simulink library "winch001_cl"  (R2022a)
settings: Solver=VariableStepAuto  StartTime=0.0  StopTime=10.0  RelTol=1e-3
undefined symbols (not defined in the file): firstOrderFilter, firstOrderFilter_ul, wnch
settings Model: Creator=jcreed2  LastModifiedBy=lhill8
settings SolverCC: AlgebraicLoopSolver=TrustRegion
settings DebuggingCC: UnconnectedInputMsg=warning  UnconnectedOutputMsg=warning  UnconnectedLineMsg=warning  SFMachineParentedDataDiag=warning  ArithmeticOperatorsInVariantConditions=warning
settings SFSimCC: CustomCodeUndefinedFunction=UseInterfaceOnly

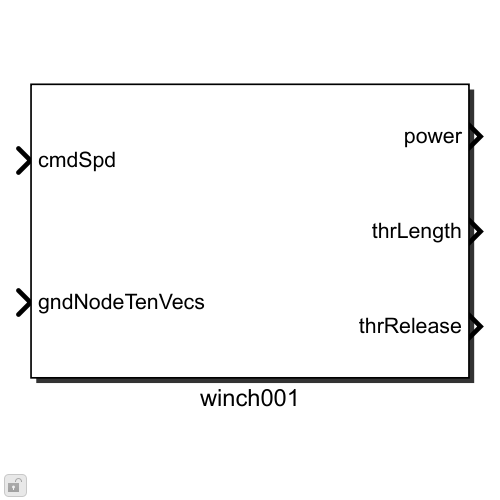
[thumbnail: Simulink's stored preview of the top-level diagram]
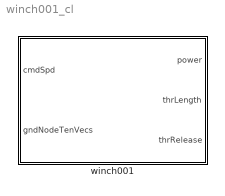
== system winch001_cl ==
  winch001 : Subsystem  VariantControl=VSS_winch_winch001

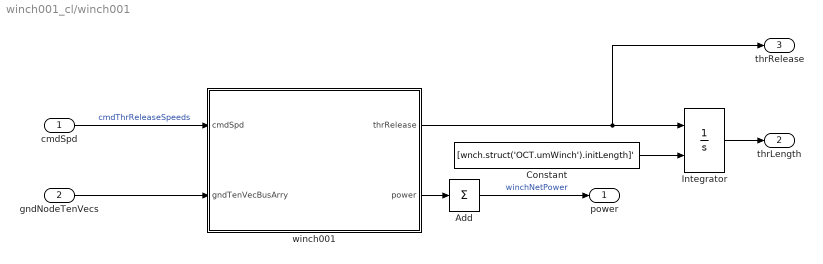
== system winch001_cl/winch001 ==
  cmdSpd : Inport
  gndNodeTenVecs : Inport  Port=2
  Add : Sum  Inputs=+
  Constant : Constant  Value=[wnch.struct('OCT.umWinch').initLength]'  VectorParams1D=off
  Integrator : Integrator  InitialConditionSource=external
  winch001 : Subsystem  mask{wnchStrct=wnch.struct('OCT.umWinch')}
      mask prompts: wnchStrct "Winch Structure"
  power : Outport  VectorParamsAs1DForOutWhenUnconnected=off
  thrLength : Outport  Port=2  VectorParamsAs1DForOutWhenUnconnected=off
  thrRelease : Outport  Port=3  VectorParamsAs1DForOutWhenUnconnected=off
  wires:
  winch001/1(thrRelease) -> Integrator/1, thrRelease/1
  Integrator/1 -> thrLength/1
  Constant/1 -> Integrator/2
  Add/1 -> power/1  "winchNetPower"
  winch001/2(power) -> Add/1
  gndNodeTenVecs/1 -> winch001/2(gndTenVecBusArry)
  cmdSpd/1 -> winch001/1(cmdSpd)  "cmdThrReleaseSpeeds"

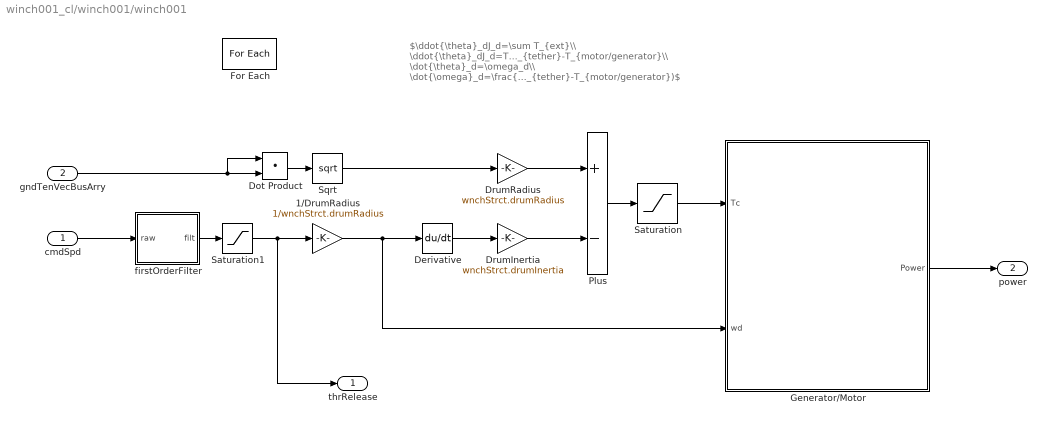
== system winch001_cl/winch001/winch001 ==
  note: $\ddot{\theta}_dJ_d=\sum T_{ext}\\ \ddot{\theta}_dJ_d=T_{tether}-T_{motor/generator}\\ \dot{\theta}_d=\omega_d\\ \dot{\omega}_d=\frac{1}{J_d}(T_{tether}-T_{motor/generator})$
  cmdSpd : Inport  Partition=on  PartitionDimension=1  PartitionWidth=1  PartitionOffset=0
  gndTenVecBusArry : Inport  Port=2  Partition=on  PartitionDimension=3  PartitionWidth=1  PartitionOffset=0
  1/DrumRadius : Gain  Gain=1/wnchStrct.drumRadius
  Derivative : Derivative
  Dot Product : DotProduct  OutDataTypeStr=Inherit: Inherit via internal rule
  DrumInertia : Gain  Gain=wnchStrct.drumInertia
  DrumRadius : Gain  Gain=wnchStrct.drumRadius
  For Each : ForEach  DisableCoverage=on  IterateSubsysMaskParameter=on  SubsysMaskParameterIterationDimension=2
  Generator/Motor : Subsystem
  Plus : Sum  Inputs=+-
  Saturation : Saturate  UpperLimit=inf  LowerLimit=0
  Saturation1 : Saturate  UpperLimit=wnchStrct.maxSpeed  LowerLimit=-wnchStrct.maxSpeed  LinearizeAsGain=off
  Sqrt : Sqrt
  firstOrderFilter : Subsystem  AncestorBlock=firstOrderFilter_ul/firstOrderFilter  TreatAsAtomicUnit=on  mask{tau=wnchStrct.timeConst, ic=wnchStrct.initReleaseRate}
      mask prompts: tau "Time Const [s]"; ic "Initial Condition"
      settings: MinAlgLoopOccurrences=on
  thrRelease : Outport  ConcatenationDimension=1  VectorParamsAs1DForOutWhenUnconnected=off
  power : Outport  Port=2  ConcatenationDimension=1  VectorParamsAs1DForOutWhenUnconnected=off
  wires:
  DrumInertia/1 -> Plus/2
  Derivative/1 -> DrumInertia/1
  DrumRadius/1 -> Plus/1
  Sqrt/1 -> DrumRadius/1
  Saturation1/1 -> 1/DrumRadius/1, thrRelease/1
  gndTenVecBusArry/1 -> Dot Product/2, Dot Product/1
  Dot Product/1 -> Sqrt/1
  Saturation/1 -> Generator/Motor/1(Tc)
  cmdSpd/1 -> firstOrderFilter/1(raw)
  1/DrumRadius/1 -> Generator/Motor/2(wd), Derivative/1
  Plus/1 -> Saturation/1
  Generator/Motor/1(Power) -> power/1
  firstOrderFilter/1(filt) -> Saturation1/1

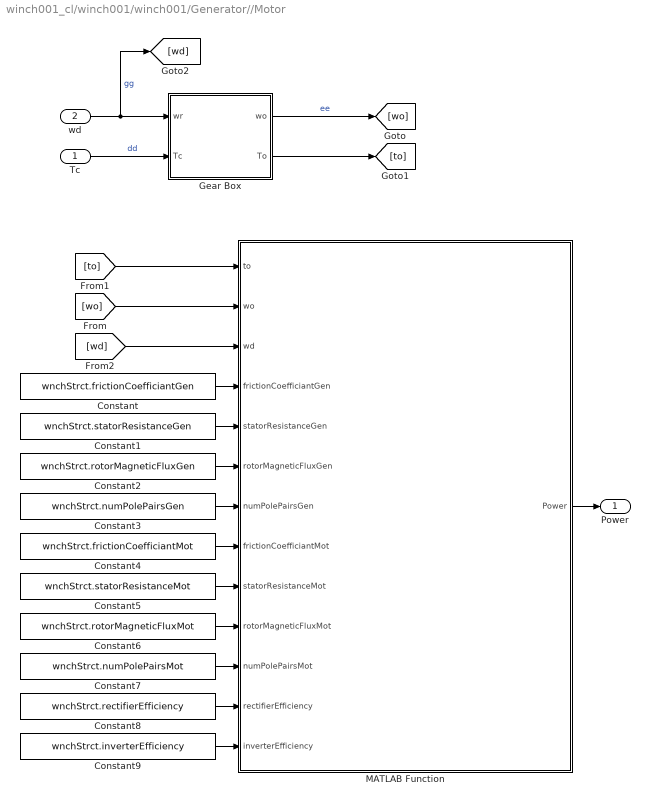
== system winch001_cl/winch001/winch001/Generator//Motor ==
  Tc : Inport
  wd : Inport  Port=2
  Constant : Constant  Value=wnchStrct.frictionCoefficiantGen
  Constant1 : Constant  Value=wnchStrct.statorResistanceGen
  Constant2 : Constant  Value=wnchStrct.rotorMagneticFluxGen
  Constant3 : Constant  Value=wnchStrct.numPolePairsGen
  Constant4 : Constant  Value=wnchStrct.frictionCoefficiantMot
  Constant5 : Constant  Value=wnchStrct.statorResistanceMot
  Constant6 : Constant  Value=wnchStrct.rotorMagneticFluxMot
  Constant7 : Constant  Value=wnchStrct.numPolePairsMot
  Constant8 : Constant  Value=wnchStrct.rectifierEfficiency
  Constant9 : Constant  Value=wnchStrct.inverterEfficiency
  Gear Box : Subsystem  mask{gfb=wnchStrct.gearRatio, Np=wnchStrct.numOfGearPairs}
      mask prompts: gfb "Gear Ratio"; Np "Number of Gear Pairs"
  MATLAB Function : MATLAB Function  TreatAsAtomicUnit=on
  Power : Outport  VectorParamsAs1DForOutWhenUnconnected=off
  wires:
  [wd] -> MATLAB Function/3(wd)
  [to] -> MATLAB Function/1(to)
  [wo] -> MATLAB Function/2(wo)
  Gear Box/2(To) -> [to]
  Gear Box/1(wo) -> [wo]  "ee"
  MATLAB Function/1(Power) -> Power/1
  Constant9/1 -> MATLAB Function/13(inverterEfficiency)
  Constant8/1 -> MATLAB Function/12(rectifierEfficiency)
  Constant7/1 -> MATLAB Function/11(numPolePairsMot)
  Constant6/1 -> MATLAB Function/10(rotorMagneticFluxMot)
  Constant5/1 -> MATLAB Function/9(statorResistanceMot)
  Constant4/1 -> MATLAB Function/8(frictionCoefficiantMot)
  Constant3/1 -> MATLAB Function/7(numPolePairsGen)
  Constant2/1 -> MATLAB Function/6(rotorMagneticFluxGen)
  Constant1/1 -> MATLAB Function/5(statorResistanceGen)
  Constant/1 -> MATLAB Function/4(frictionCoefficiantGen)
  wd/1 -> Gear Box/1(wr), [wd]  "gg"
  Tc/1 -> Gear Box/2(Tc)  "dd"

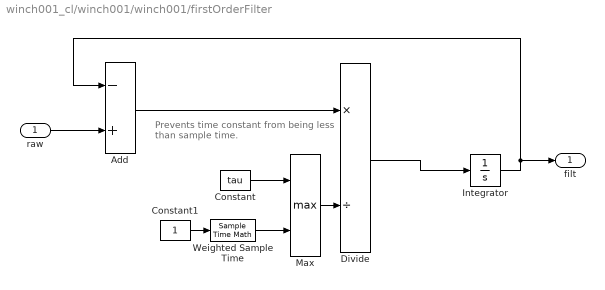
== system winch001_cl/winch001/winch001/firstOrderFilter ==
  note: Prevents time constant from
      | being less than sample time.
  raw : Inport
  Add : Sum  Inputs=-+
  Constant : Constant  Value=tau
  Constant1 : Constant
  Divide : Product  Inputs=*/
  Integrator : Integrator  InitialCondition=ic
  Max : MinMax  Function=max  Inputs=2
  Weighted Sample Time : SampleTimeMath  TsampMathOp=Ts Only
  filt : Outport  VectorParamsAs1DForOutWhenUnconnected=off
  wires:
  raw/1 -> Add/2
  Add/1 -> Divide/1
  Max/1 -> Divide/2
  Constant/1 -> Max/1
  Constant1/1 -> Weighted Sample Time/1
  Weighted Sample Time/1 -> Max/2
  Divide/1 -> Integrator/1
  Integrator/1 -> Add/1, filt/1

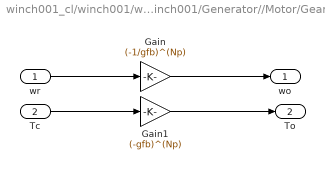
== system winch001_cl/winch001/winch001/Generator//Motor/Gear Box ==
  wr : Inport
  Tc : Inport  Port=2
  Gain : Gain  Gain=(-1/gfb)^(Np)
  Gain1 : Gain  Gain=(-gfb)^(Np)
  wo : Outport  VectorParamsAs1DForOutWhenUnconnected=off
  To : Outport  Port=2  VectorParamsAs1DForOutWhenUnconnected=off
  wires:
  wr/1 -> Gain/1
  Gain/1 -> wo/1
  Tc/1 -> Gain1/1
  Gain1/1 -> To/1

== matlab function winch001_cl/winch001/winch001/Generator//Motor/MATLAB Function ==
  data: to input; Power output; wo input; wd input; frictionCoefficiantGen input; statorResistanceGen input; rotorMagneticFluxGen input; numPolePairsGen input; frictionCoefficiantMot input; statorResistanceMot input; rotorMagneticFluxMot input; numPolePairsMot input; rectifierEfficiency input; inverterEfficiency input
function Power = fcn(to,wo,wd,frictionCoefficiantGen,statorResistanceGen,rotorMagneticFluxGen,numPolePairsGen,frictionCoefficiantMot,statorResistanceMot,rotorMagneticFluxMot,numPolePairsMot,rectifierEfficiency,inverterEfficiency)


Power = 0;

switch sign(wd)
    case 1
        
        wdAbs = abs(wo);
        
        Tf = frictionCoefficiantGen*wdAbs;
        
        eta = (to*wdAbs)/(2*statorResistanceGen*to^2/(3*rotorMagneticFluxGen^2*numPolePairsGen^2)+4*statorResistanceGen*Tf*to/(3*rotorMagneticFluxGen^2*numPolePairsGen^2)+wdAbs*to+...
            2*statorResistanceGen*Tf^2/(3*rotorMagneticFluxGen^2*numPolePairsGen^2)+wdAbs*Tf);
        
        if eta >1
            eta = 1;
        end
        if eta <0
            eta = 0;
        end
        
        int = to*wo;
        Power = eta*int*rectifierEfficiency;
   
    case -1
        
        
        toAbs = abs(to);
        wdAbs = abs(wo);
        
        
        Tf = frictionCoefficiantMot*wdAbs;
        
        eta = (toAbs*wdAbs)/(2*statorResistanceMot*toAbs^2/(3*rotorMagneticFluxMot^2*numPolePairsMot^2)+4*statorResistanceMot*Tf*toAbs/(3*rotorMagneticFluxMot^2*numPolePairsMot^2)+wdAbs*toAbs+...
            2*statorResistanceMot*Tf^2/(3*rotorMagneticFluxMot^2*numPolePairsMot^2)+wdAbs*Tf);
        
        
        
        
        
        if eta >1
            eta = 1;
        end
        if eta <0
            eta = 0;
        end
        
        int = to*wo;
        Power = (int/eta)*(1/inverterEfficiency);
        
end
if isnan(Power)
    x = 2;
end
end
